simulink model "accelerometerSwithcAndDisplay"  (R2016b)
settings: Solver=FixedStepAuto  StartTime=0.0  StopTime=inf  RelTol=1e-3
libraries: androidlib x3
settings Model: SimulationMode=external  Creator=vibek  LastModifiedBy=vibek
settings OptimizationCC: MaxStackSize=64
settings DebuggingCC: ParameterTunabilityLossMsg=error
settings HardwareCC: ProdBitPerPointer=32  ProdBitPerSizeT=32  ProdBitPerPtrDiffT=32  ProdLargestAtomicInteger=Long  ProdLargestAtomicFloat=Double  ProdWordSize=32  ProdHWDeviceType=ARM Compatible->ARM Cortex  UseEmbeddedCoderFeatures=off  UseSimulinkCoderFeatures=off
settings RTWCC: SystemTargetFile=ert.tlc  HardwareBoard=Android Device  TLCOptions="-aInlineSetEventsForThisBaseRateFcn=TLC_FALSE -aSuppressMultiTaskScheduler=TLC_FALSE  -aRateBasedStepFcn=0"  TemplateMakefile=ert_default_tmf  Description=Embedded Coder  GenerateReport=on  Toolchain=Android SDK/NDK Tools  IncludeHyperlinkInReport=on  LaunchReport=on  GenerateTraceInfo=on  GenerateTraceReport=on  GenerateTraceReportSl=on  GenerateTraceReportSf=on  GenerateTraceReportEml=on
settings CodeAppCC: ForceParamTrailComments=on  IgnoreCustomStorageClasses=off  OperatorAnnotations=on  SimulinkDataObjDesc=on  SFDataObjDesc=on  MATLABFcnDesc=on  InsertBlockDesc=on  MATLABSourceComments=on
settings ERTTargetCC: SupportNonInlinedSFcns=on

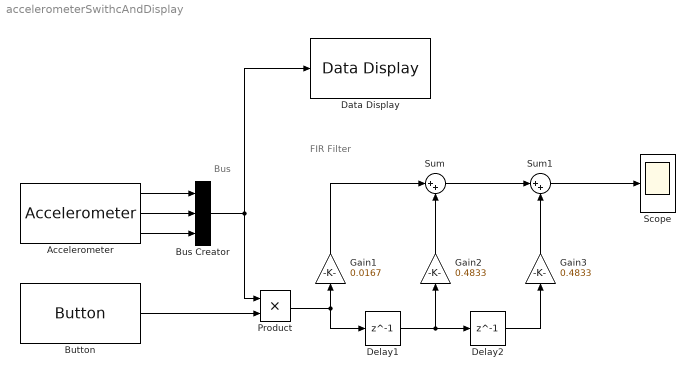
== system accelerometerSwithcAndDisplay ==
  note: FIR Filter
  note: Bus
  Accelerometer : androidlib/Accelerometer  OutputVector=off  SampleTime=0.1  BlockPlatform=Android
  Bus Creator : BusCreator  Inputs=3
  Button : androidlib/Button  ButtonState=Not pressed  ButtonId=accelerometer_Button  State=off  SampleTime=0.1  BlockPlatform=Android
  Data Display : androidlib/Data Display  DataDisplayId=accelerometer_Data_Display  Format=Float  Precision=6  SimulateUsing=Code generation  blockPlatform=Android
  Delay1 : Delay  DelayLength=1
  Delay2 : Delay  DelayLength=1
  Gain1 : Gain  Gain=0.0167
  Gain2 : Gain  Gain=0.4833
  Gain3 : Gain  Gain=0.4833
  Product : Product
  Scope : Scope
  Sum : Sum  Inputs=|++
  Sum1 : Sum  Inputs=|++
  wires:
  Gain1/1 -> Sum/1
  Gain2/1 -> Sum/2
  Delay1/1 -> Delay2/1, Gain2/1
  Delay2/1 -> Gain3/1
  Sum/1 -> Sum1/1
  Gain3/1 -> Sum1/2
  Sum1/1 -> Scope/1
  Accelerometer/3 -> Bus Creator/3
  Accelerometer/1 -> Bus Creator/1
  Accelerometer/2 -> Bus Creator/2
  Bus Creator/1 -> Data Display/1, Product/1
  Button/1 -> Product/2
  Product/1 -> Delay1/1, Gain1/1
